simulink model "FRNmodel_IMHRC"  (Simulink 7.9)
settings: Solver=VariableStepDiscrete  StartTime=0.0  StopTime=100.0  RelTol=1e-3
libraries: simeventslib x30
(part 1 of 3)
settings Model: Creator=tsprock3  LastModifiedBy=tsprock3
settings DebuggingCC: SimStateOlderReleaseMsg=warning

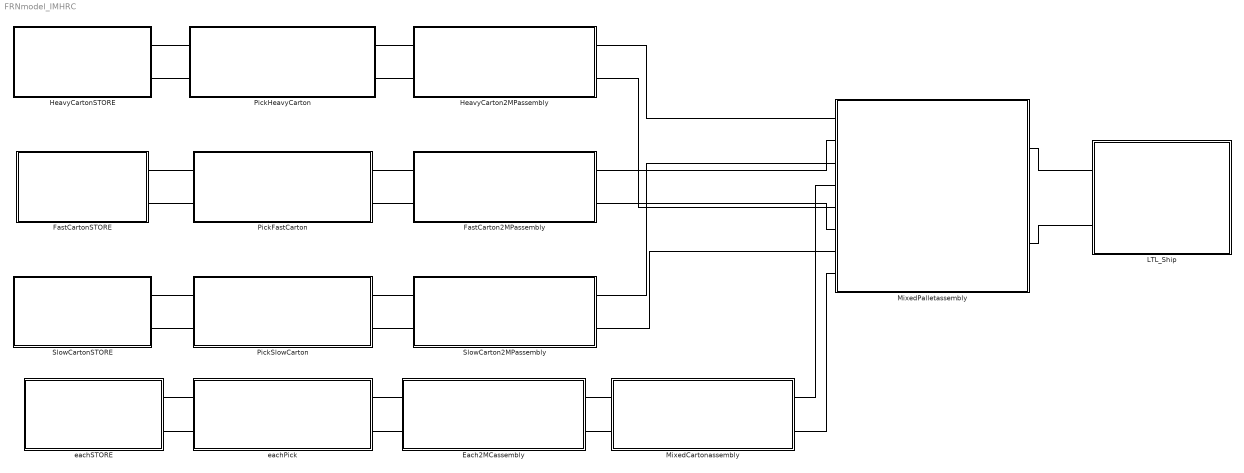
== system FRNmodel_IMHRC ==
  Each2MCassembly : Subsystem
  FastCarton2MPassembly : Subsystem
  FastCartonSTORE : Subsystem
  HeavyCarton2MPassembly : Subsystem
  HeavyCartonSTORE : Subsystem
  LTL_Ship : Subsystem
  MixedCartonassembly : Subsystem
  MixedPalletassembly : Subsystem
  PickFastCarton : Subsystem
  PickHeavyCarton : Subsystem
  PickSlowCarton : Subsystem
  SlowCarton2MPassembly : Subsystem
  SlowCartonSTORE : Subsystem
  eachPick : Subsystem
  eachSTORE : Subsystem
  connections:
  HeavyCartonSTORE/RConn1 -- PickHeavyCarton/LConn1
  FastCartonSTORE/RConn1 -- PickFastCarton/LConn1
  SlowCartonSTORE/RConn1 -- PickSlowCarton/LConn1
  PickHeavyCarton/RConn1 -- HeavyCarton2MPassembly/LConn1
  PickFastCarton/RConn1 -- FastCarton2MPassembly/LConn1
  PickSlowCarton/RConn1 -- SlowCarton2MPassembly/LConn1
  HeavyCarton2MPassembly/RConn1 -- MixedPalletassembly/LConn1
  MixedPalletassembly/RConn1 -- LTL_Ship/LConn1
  FastCarton2MPassembly/RConn1 -- MixedPalletassembly/LConn2
  SlowCarton2MPassembly/RConn1 -- MixedPalletassembly/LConn3
  HeavyCartonSTORE/RConn2 -- PickHeavyCarton/LConn2
  PickFastCarton/LConn2 -- FastCartonSTORE/RConn2
  PickSlowCarton/LConn2 -- SlowCartonSTORE/RConn2
  PickSlowCarton/RConn2 -- SlowCarton2MPassembly/LConn2
  PickFastCarton/RConn2 -- FastCarton2MPassembly/LConn2
  HeavyCarton2MPassembly/LConn2 -- PickHeavyCarton/RConn2
  MixedPalletassembly/LConn5 -- HeavyCarton2MPassembly/RConn2
  MixedPalletassembly/LConn6 -- FastCarton2MPassembly/RConn2
  MixedPalletassembly/LConn7 -- SlowCarton2MPassembly/RConn2
  LTL_Ship/LConn2 -- MixedPalletassembly/RConn2
  Each2MCassembly/RConn1 -- MixedCartonassembly/LConn1
  eachSTORE/RConn1 -- eachPick/LConn1
  eachPick/RConn1 -- Each2MCassembly/LConn1
  eachPick/LConn2 -- eachSTORE/RConn2
  eachPick/RConn2 -- Each2MCassembly/LConn2
  Each2MCassembly/RConn2 -- MixedCartonassembly/LConn2
  MixedPalletassembly/LConn8 -- MixedCartonassembly/RConn2
  MixedPalletassembly/LConn4 -- MixedCartonassembly/RConn1

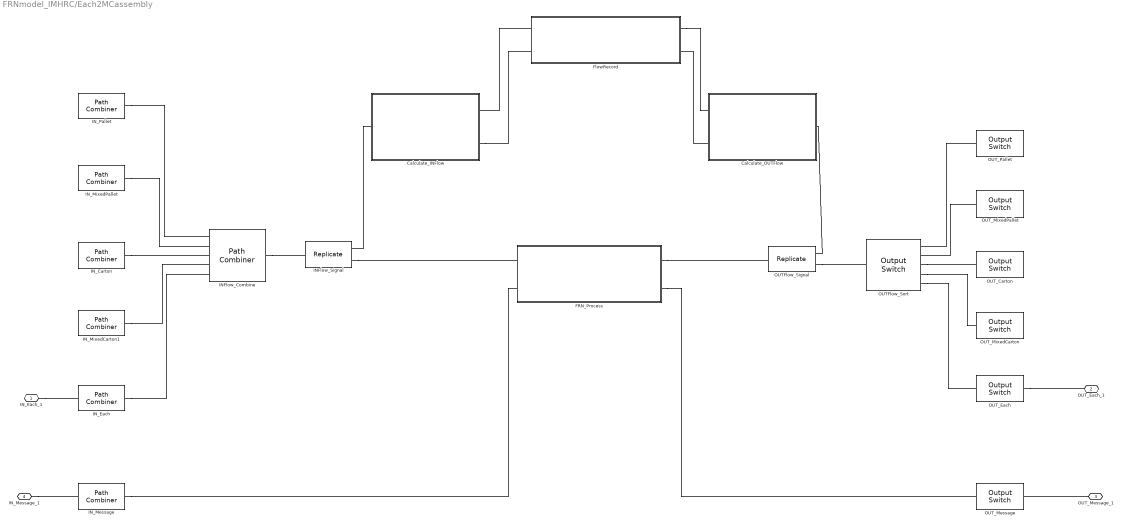
== system FRNmodel_IMHRC/Each2MCassembly ==
  Calculate_INFlow : Subsystem
  Calculate_OUTFlow : Subsystem
  FRN_Process : Subsystem
  FlowRecord : Subsystem
  INFlow_Combine : PathCombiner  NumberInputPorts=5
  INFlow_Signal : Replicate  NumberOutputPorts=2
  IN_Carton : PathCombiner  NumberInputPorts=1
  IN_Each : PathCombiner  NumberInputPorts=1
  IN_Message : PathCombiner  NumberInputPorts=1
  IN_MixedCarton1 : PathCombiner  NumberInputPorts=1
  IN_MixedPallet : PathCombiner  NumberInputPorts=1
  IN_Pallet : PathCombiner  NumberInputPorts=1
  OUTFlow_Signal : Replicate  NumberOutputPorts=2
  OUTFlow_Sort : OutputSwitch  NumberOutputPorts=5  SwitchingCriterion=From attribute  AttributeName=UoH
  OUT_Carton : OutputSwitch  NumberOutputPorts=1
  OUT_Each : OutputSwitch  NumberOutputPorts=1
  OUT_Message : OutputSwitch  NumberOutputPorts=1
  OUT_MixedCarton : OutputSwitch  NumberOutputPorts=1
  OUT_MixedPallet : OutputSwitch  NumberOutputPorts=1
  OUT_Pallet : OutputSwitch  NumberOutputPorts=1
  IN_Each_1 : PMIOPort  Port=1  Side=Left
  OUT_Each_1 : PMIOPort  Port=2  Side=Right
  OUT_Message_1 : PMIOPort  Port=3  Side=Left
  IN_Message_1 : PMIOPort  Port=4  Side=Right
  connections:
  Calculate_INFlow/LConn1 -- INFlow_Signal/RConn1
  FlowRecord/RConn1 -- Calculate_INFlow/RConn1
  Calculate_INFlow/RConn2 -- FlowRecord/RConn2
  FlowRecord/LConn1 -- Calculate_OUTFlow/LConn1
  Calculate_OUTFlow/LConn2 -- FlowRecord/LConn2
  INFlow_Signal/RConn2 -- FRN_Process/LConn1
  FRN_Process/RConn1 -- OUTFlow_Signal/LConn1
  OUTFlow_Signal/RConn1 -- Calculate_OUTFlow/RConn1
  INFlow_Combine/RConn1 -- INFlow_Signal/LConn1
  IN_Pallet/RConn1 -- INFlow_Combine/LConn1
  IN_Carton/RConn1 -- INFlow_Combine/LConn3
  IN_Each/RConn1 -- INFlow_Combine/LConn5
  OUTFlow_Signal/RConn2 -- OUTFlow_Sort/LConn1
  OUT_Pallet/LConn1 -- OUTFlow_Sort/RConn1
  OUTFlow_Sort/RConn3 -- OUT_Carton/LConn1
  OUTFlow_Sort/RConn5 -- OUT_Each/LConn1
  IN_Message_1/RConn1 -- IN_Message/LConn1
  OUT_Message_1/RConn1 -- OUT_Message/RConn1
  IN_Message/RConn1 -- FRN_Process/LConn2
  FRN_Process/RConn2 -- OUT_Message/LConn1
  OUT_MixedPallet/LConn1 -- OUTFlow_Sort/RConn2
  OUTFlow_Sort/RConn4 -- OUT_MixedCarton/LConn1
  IN_MixedPallet/RConn1 -- INFlow_Combine/LConn2
  IN_MixedCarton1/RConn1 -- INFlow_Combine/LConn4
  IN_Each_1/RConn1 -- IN_Each/LConn1
  OUT_Each/RConn1 -- OUT_Each_1/RConn1

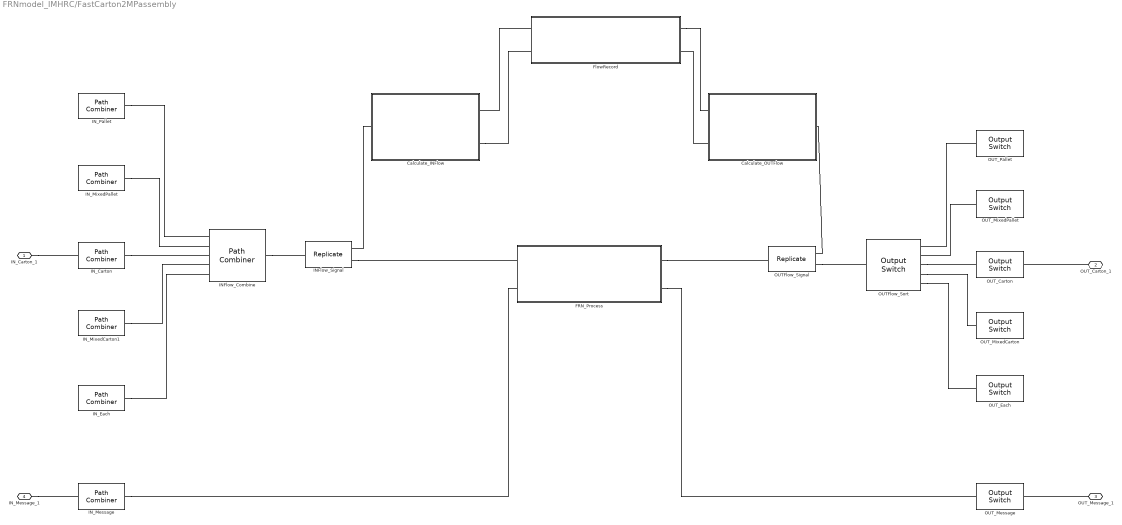
== system FRNmodel_IMHRC/FastCarton2MPassembly ==
  Calculate_INFlow : Subsystem
  Calculate_OUTFlow : Subsystem
  FRN_Process : Subsystem
  FlowRecord : Subsystem
  INFlow_Combine : PathCombiner  NumberInputPorts=5
  INFlow_Signal : Replicate  NumberOutputPorts=2
  IN_Carton : PathCombiner  NumberInputPorts=1
  IN_Each : PathCombiner  NumberInputPorts=1
  IN_Message : PathCombiner  NumberInputPorts=1
  IN_MixedCarton1 : PathCombiner  NumberInputPorts=1
  IN_MixedPallet : PathCombiner  NumberInputPorts=1
  IN_Pallet : PathCombiner  NumberInputPorts=1
  OUTFlow_Signal : Replicate  NumberOutputPorts=2
  OUTFlow_Sort : OutputSwitch  NumberOutputPorts=5  SwitchingCriterion=From attribute  AttributeName=UoH
  OUT_Carton : OutputSwitch  NumberOutputPorts=1
  OUT_Each : OutputSwitch  NumberOutputPorts=1
  OUT_Message : OutputSwitch  NumberOutputPorts=1
  OUT_MixedCarton : OutputSwitch  NumberOutputPorts=1
  OUT_MixedPallet : OutputSwitch  NumberOutputPorts=1
  OUT_Pallet : OutputSwitch  NumberOutputPorts=1
  IN_Carton_1 : PMIOPort  Port=1  Side=Left
  OUT_Carton_1 : PMIOPort  Port=2  Side=Right
  OUT_Message_1 : PMIOPort  Port=3  Side=Left
  IN_Message_1 : PMIOPort  Port=4  Side=Right
  connections:
  Calculate_INFlow/LConn1 -- INFlow_Signal/RConn1
  FlowRecord/RConn1 -- Calculate_INFlow/RConn1
  Calculate_INFlow/RConn2 -- FlowRecord/RConn2
  FlowRecord/LConn1 -- Calculate_OUTFlow/LConn1
  Calculate_OUTFlow/LConn2 -- FlowRecord/LConn2
  INFlow_Signal/RConn2 -- FRN_Process/LConn1
  FRN_Process/RConn1 -- OUTFlow_Signal/LConn1
  OUTFlow_Signal/RConn1 -- Calculate_OUTFlow/RConn1
  INFlow_Combine/RConn1 -- INFlow_Signal/LConn1
  IN_Pallet/RConn1 -- INFlow_Combine/LConn1
  IN_Carton_1/RConn1 -- IN_Carton/LConn1
  IN_Carton/RConn1 -- INFlow_Combine/LConn3
  IN_Each/RConn1 -- INFlow_Combine/LConn5
  OUTFlow_Signal/RConn2 -- OUTFlow_Sort/LConn1
  OUT_Pallet/LConn1 -- OUTFlow_Sort/RConn1
  OUT_Carton_1/RConn1 -- OUT_Carton/RConn1
  OUTFlow_Sort/RConn3 -- OUT_Carton/LConn1
  OUTFlow_Sort/RConn5 -- OUT_Each/LConn1
  IN_Message_1/RConn1 -- IN_Message/LConn1
  OUT_Message_1/RConn1 -- OUT_Message/RConn1
  IN_Message/RConn1 -- FRN_Process/LConn2
  FRN_Process/RConn2 -- OUT_Message/LConn1
  OUT_MixedPallet/LConn1 -- OUTFlow_Sort/RConn2
  OUTFlow_Sort/RConn4 -- OUT_MixedCarton/LConn1
  IN_MixedPallet/RConn1 -- INFlow_Combine/LConn2
  IN_MixedCarton1/RConn1 -- INFlow_Combine/LConn4

== system FRNmodel_IMHRC/FastCartonSTORE ==
  Calculate_INFlow : Subsystem
  Calculate_OUTFlow : Subsystem
  FRN_Process : Subsystem
  FlowRecord : Subsystem
  INFlow_Combine : PathCombiner  NumberInputPorts=5
  INFlow_Signal : Replicate  NumberOutputPorts=2
  IN_Carton : PathCombiner  NumberInputPorts=1
  IN_Each : PathCombiner  NumberInputPorts=1
  IN_Message : PathCombiner  NumberInputPorts=1
  IN_MixedCarton1 : PathCombiner  NumberInputPorts=1
  IN_MixedPallet : PathCombiner  NumberInputPorts=1
  IN_Pallet : PathCombiner  NumberInputPorts=1
  OUTFlow_Signal : Replicate  NumberOutputPorts=2
  OUTFlow_Sort : OutputSwitch  NumberOutputPorts=5  SwitchingCriterion=From attribute  AttributeName=UoH
  OUT_Carton : OutputSwitch  NumberOutputPorts=1
  OUT_Each : OutputSwitch  NumberOutputPorts=1
  OUT_Message : OutputSwitch  NumberOutputPorts=1
  OUT_MixedCarton : OutputSwitch  NumberOutputPorts=1
  OUT_MixedPallet : OutputSwitch  NumberOutputPorts=1
  OUT_Pallet : OutputSwitch  NumberOutputPorts=1
  OUT_Carton_1 : PMIOPort  Port=1  Side=Right
  IN_Message_1 : PMIOPort  Port=2  Side=Right
  connections:
  Calculate_INFlow/LConn1 -- INFlow_Signal/RConn1
  FlowRecord/RConn1 -- Calculate_INFlow/RConn1
  Calculate_INFlow/RConn2 -- FlowRecord/RConn2
  FlowRecord/LConn1 -- Calculate_OUTFlow/LConn1
  Calculate_OUTFlow/LConn2 -- FlowRecord/LConn2
  INFlow_Signal/RConn2 -- FRN_Process/LConn1
  FRN_Process/RConn1 -- OUTFlow_Signal/LConn1
  OUTFlow_Signal/RConn1 -- Calculate_OUTFlow/RConn1
  INFlow_Combine/RConn1 -- INFlow_Signal/LConn1
  IN_Pallet/RConn1 -- INFlow_Combine/LConn1
  IN_Carton/RConn1 -- INFlow_Combine/LConn3
  IN_Each/RConn1 -- INFlow_Combine/LConn5
  OUTFlow_Signal/RConn2 -- OUTFlow_Sort/LConn1
  OUT_Pallet/LConn1 -- OUTFlow_Sort/RConn1
  OUT_Carton_1/RConn1 -- OUT_Carton/RConn1
  OUTFlow_Sort/RConn3 -- OUT_Carton/LConn1
  OUTFlow_Sort/RConn5 -- OUT_Each/LConn1
  IN_Message_1/RConn1 -- IN_Message/LConn1
  IN_Message/RConn1 -- FRN_Process/LConn2
  FRN_Process/RConn2 -- OUT_Message/LConn1
  OUT_MixedPallet/LConn1 -- OUTFlow_Sort/RConn2
  OUTFlow_Sort/RConn4 -- OUT_MixedCarton/LConn1
  IN_MixedPallet/RConn1 -- INFlow_Combine/LConn2
  IN_MixedCarton1/RConn1 -- INFlow_Combine/LConn4

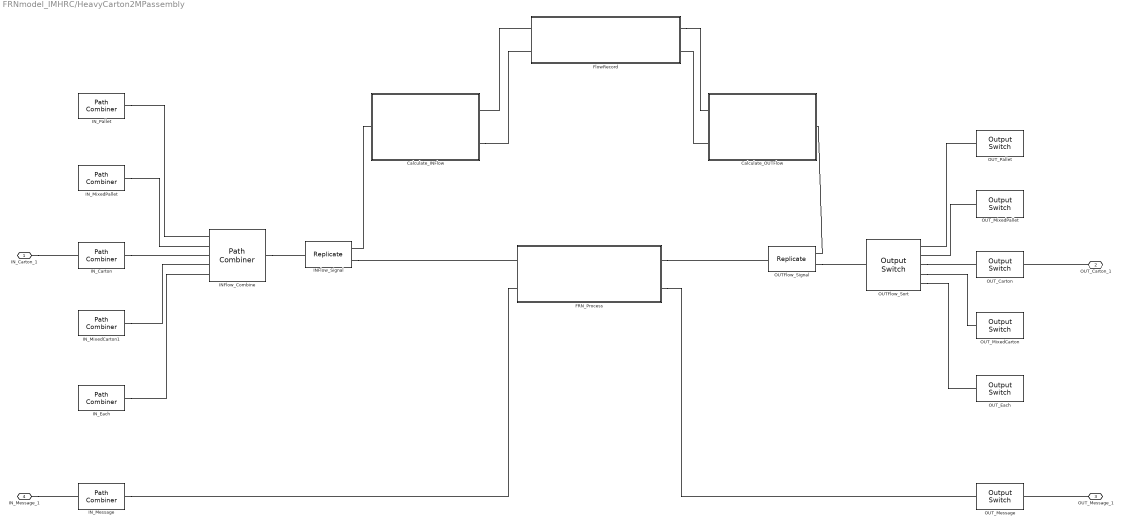
== system FRNmodel_IMHRC/HeavyCarton2MPassembly ==
  Calculate_INFlow : Subsystem
  Calculate_OUTFlow : Subsystem
  FRN_Process : Subsystem
  FlowRecord : Subsystem
  INFlow_Combine : PathCombiner  NumberInputPorts=5
  INFlow_Signal : Replicate  NumberOutputPorts=2
  IN_Carton : PathCombiner  NumberInputPorts=1
  IN_Each : PathCombiner  NumberInputPorts=1
  IN_Message : PathCombiner  NumberInputPorts=1
  IN_MixedCarton1 : PathCombiner  NumberInputPorts=1
  IN_MixedPallet : PathCombiner  NumberInputPorts=1
  IN_Pallet : PathCombiner  NumberInputPorts=1
  OUTFlow_Signal : Replicate  NumberOutputPorts=2
  OUTFlow_Sort : OutputSwitch  NumberOutputPorts=5  SwitchingCriterion=From attribute  AttributeName=UoH
  OUT_Carton : OutputSwitch  NumberOutputPorts=1
  OUT_Each : OutputSwitch  NumberOutputPorts=1
  OUT_Message : OutputSwitch  NumberOutputPorts=1
  OUT_MixedCarton : OutputSwitch  NumberOutputPorts=1
  OUT_MixedPallet : OutputSwitch  NumberOutputPorts=1
  OUT_Pallet : OutputSwitch  NumberOutputPorts=1
  IN_Carton_1 : PMIOPort  Port=1  Side=Left
  OUT_Carton_1 : PMIOPort  Port=2  Side=Right
  OUT_Message_1 : PMIOPort  Port=3  Side=Left
  IN_Message_1 : PMIOPort  Port=4  Side=Right
  connections:
  Calculate_INFlow/LConn1 -- INFlow_Signal/RConn1
  FlowRecord/RConn1 -- Calculate_INFlow/RConn1
  Calculate_INFlow/RConn2 -- FlowRecord/RConn2
  FlowRecord/LConn1 -- Calculate_OUTFlow/LConn1
  Calculate_OUTFlow/LConn2 -- FlowRecord/LConn2
  INFlow_Signal/RConn2 -- FRN_Process/LConn1
  FRN_Process/RConn1 -- OUTFlow_Signal/LConn1
  OUTFlow_Signal/RConn1 -- Calculate_OUTFlow/RConn1
  INFlow_Combine/RConn1 -- INFlow_Signal/LConn1
  IN_Pallet/RConn1 -- INFlow_Combine/LConn1
  IN_Carton_1/RConn1 -- IN_Carton/LConn1
  IN_Carton/RConn1 -- INFlow_Combine/LConn3
  IN_Each/RConn1 -- INFlow_Combine/LConn5
  OUTFlow_Signal/RConn2 -- OUTFlow_Sort/LConn1
  OUT_Pallet/LConn1 -- OUTFlow_Sort/RConn1
  OUT_Carton_1/RConn1 -- OUT_Carton/RConn1
  OUTFlow_Sort/RConn3 -- OUT_Carton/LConn1
  OUTFlow_Sort/RConn5 -- OUT_Each/LConn1
  IN_Message_1/RConn1 -- IN_Message/LConn1
  OUT_Message_1/RConn1 -- OUT_Message/RConn1
  IN_Message/RConn1 -- FRN_Process/LConn2
  FRN_Process/RConn2 -- OUT_Message/LConn1
  OUT_MixedPallet/LConn1 -- OUTFlow_Sort/RConn2
  OUTFlow_Sort/RConn4 -- OUT_MixedCarton/LConn1
  IN_MixedPallet/RConn1 -- INFlow_Combine/LConn2
  IN_MixedCarton1/RConn1 -- INFlow_Combine/LConn4

== system FRNmodel_IMHRC/HeavyCartonSTORE ==
  Calculate_INFlow : Subsystem
  Calculate_OUTFlow : Subsystem
  FRN_Process : Subsystem
  FlowRecord : Subsystem
  INFlow_Combine : PathCombiner  NumberInputPorts=5
  INFlow_Signal : Replicate  NumberOutputPorts=2
  IN_Carton : PathCombiner  NumberInputPorts=1
  IN_Each : PathCombiner  NumberInputPorts=1
  IN_Message : PathCombiner  NumberInputPorts=1
  IN_MixedCarton1 : PathCombiner  NumberInputPorts=1
  IN_MixedPallet : PathCombiner  NumberInputPorts=1
  IN_Pallet : PathCombiner  NumberInputPorts=1
  OUTFlow_Signal : Replicate  NumberOutputPorts=2
  OUTFlow_Sort : OutputSwitch  NumberOutputPorts=5  SwitchingCriterion=From attribute  AttributeName=UoH
  OUT_Carton : OutputSwitch  NumberOutputPorts=1
  OUT_Each : OutputSwitch  NumberOutputPorts=1
  OUT_Message : OutputSwitch  NumberOutputPorts=1
  OUT_MixedCarton : OutputSwitch  NumberOutputPorts=1
  OUT_MixedPallet : OutputSwitch  NumberOutputPorts=1
  OUT_Pallet : OutputSwitch  NumberOutputPorts=1
  OUT_Carton_1 : PMIOPort  Port=1  Side=Right
  IN_Message_1 : PMIOPort  Port=2  Side=Right
  connections:
  Calculate_INFlow/LConn1 -- INFlow_Signal/RConn1
  FlowRecord/RConn1 -- Calculate_INFlow/RConn1
  Calculate_INFlow/RConn2 -- FlowRecord/RConn2
  FlowRecord/LConn1 -- Calculate_OUTFlow/LConn1
  Calculate_OUTFlow/LConn2 -- FlowRecord/LConn2
  INFlow_Signal/RConn2 -- FRN_Process/LConn1
  FRN_Process/RConn1 -- OUTFlow_Signal/LConn1
  OUTFlow_Signal/RConn1 -- Calculate_OUTFlow/RConn1
  INFlow_Combine/RConn1 -- INFlow_Signal/LConn1
  IN_Pallet/RConn1 -- INFlow_Combine/LConn1
  IN_Carton/RConn1 -- INFlow_Combine/LConn3
  IN_Each/RConn1 -- INFlow_Combine/LConn5
  OUTFlow_Signal/RConn2 -- OUTFlow_Sort/LConn1
  OUT_Pallet/LConn1 -- OUTFlow_Sort/RConn1
  OUT_Carton_1/RConn1 -- OUT_Carton/RConn1
  OUTFlow_Sort/RConn3 -- OUT_Carton/LConn1
  OUTFlow_Sort/RConn5 -- OUT_Each/LConn1
  IN_Message_1/RConn1 -- IN_Message/LConn1
  IN_Message/RConn1 -- FRN_Process/LConn2
  FRN_Process/RConn2 -- OUT_Message/LConn1
  OUT_MixedPallet/LConn1 -- OUTFlow_Sort/RConn2
  OUTFlow_Sort/RConn4 -- OUT_MixedCarton/LConn1
  IN_MixedPallet/RConn1 -- INFlow_Combine/LConn2
  IN_MixedCarton1/RConn1 -- INFlow_Combine/LConn4

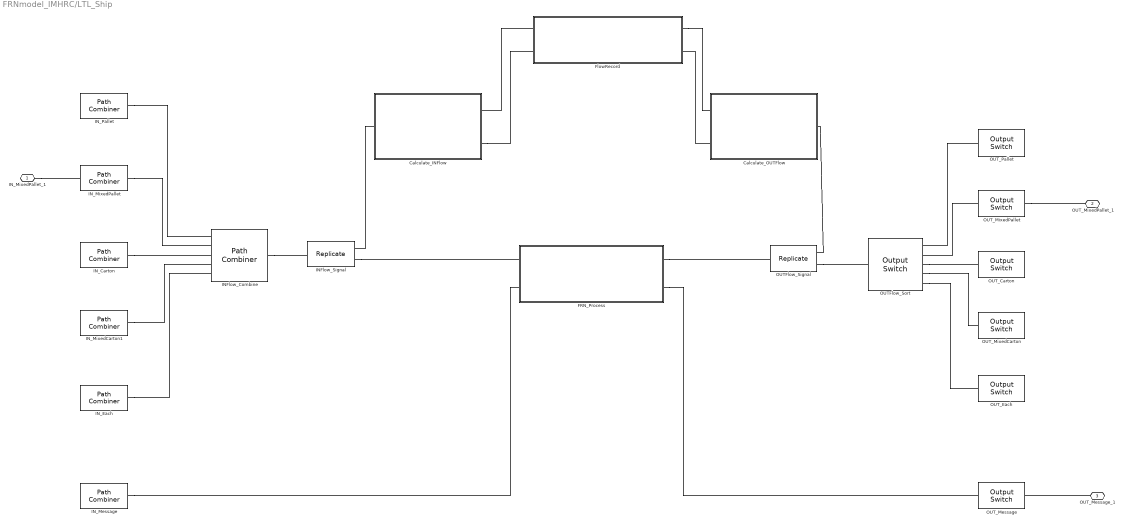
== system FRNmodel_IMHRC/LTL_Ship ==
  Calculate_INFlow : Subsystem
  Calculate_OUTFlow : Subsystem
  FRN_Process : Subsystem
  FlowRecord : Subsystem
  INFlow_Combine : PathCombiner  NumberInputPorts=5
  INFlow_Signal : Replicate  NumberOutputPorts=2
  IN_Carton : PathCombiner  NumberInputPorts=1
  IN_Each : PathCombiner  NumberInputPorts=1
  IN_Message : PathCombiner  NumberInputPorts=1
  IN_MixedCarton1 : PathCombiner  NumberInputPorts=1
  IN_MixedPallet : PathCombiner  NumberInputPorts=1
  IN_Pallet : PathCombiner  NumberInputPorts=1
  OUTFlow_Signal : Replicate  NumberOutputPorts=2
  OUTFlow_Sort : OutputSwitch  NumberOutputPorts=5  SwitchingCriterion=From attribute  AttributeName=UoH
  OUT_Carton : OutputSwitch  NumberOutputPorts=1
  OUT_Each : OutputSwitch  NumberOutputPorts=1
  OUT_Message : OutputSwitch  NumberOutputPorts=1
  OUT_MixedCarton : OutputSwitch  NumberOutputPorts=1
  OUT_MixedPallet : OutputSwitch  NumberOutputPorts=1
  OUT_Pallet : OutputSwitch  NumberOutputPorts=1
  IN_MixedPallet_1 : PMIOPort  Port=1  Side=Left
  OUT_MixedPallet_1 : PMIOPort  Port=2  Side=Right
  OUT_Message_1 : PMIOPort  Port=3  Side=Left
  connections:
  Calculate_INFlow/LConn1 -- INFlow_Signal/RConn1
  FlowRecord/RConn1 -- Calculate_INFlow/RConn1
  Calculate_INFlow/RConn2 -- FlowRecord/RConn2
  FlowRecord/LConn1 -- Calculate_OUTFlow/LConn1
  Calculate_OUTFlow/LConn2 -- FlowRecord/LConn2
  INFlow_Signal/RConn2 -- FRN_Process/LConn1
  FRN_Process/RConn1 -- OUTFlow_Signal/LConn1
  OUTFlow_Signal/RConn1 -- Calculate_OUTFlow/RConn1
  INFlow_Combine/RConn1 -- INFlow_Signal/LConn1
  IN_Pallet/RConn1 -- INFlow_Combine/LConn1
  IN_Carton/RConn1 -- INFlow_Combine/LConn3
  IN_Each/RConn1 -- INFlow_Combine/LConn5
  OUTFlow_Signal/RConn2 -- OUTFlow_Sort/LConn1
  OUT_Pallet/LConn1 -- OUTFlow_Sort/RConn1
  OUTFlow_Sort/RConn3 -- OUT_Carton/LConn1
  OUTFlow_Sort/RConn5 -- OUT_Each/LConn1
  OUT_Message_1/RConn1 -- OUT_Message/RConn1
  IN_Message/RConn1 -- FRN_Process/LConn2
  FRN_Process/RConn2 -- OUT_Message/LConn1
  OUT_MixedPallet/LConn1 -- OUTFlow_Sort/RConn2
  OUTFlow_Sort/RConn4 -- OUT_MixedCarton/LConn1
  IN_MixedPallet/RConn1 -- INFlow_Combine/LConn2
  IN_MixedPallet_1/RConn1 -- IN_MixedPallet/LConn1
  IN_MixedCarton1/RConn1 -- INFlow_Combine/LConn4
  OUT_MixedPallet/RConn1 -- OUT_MixedPallet_1/RConn1

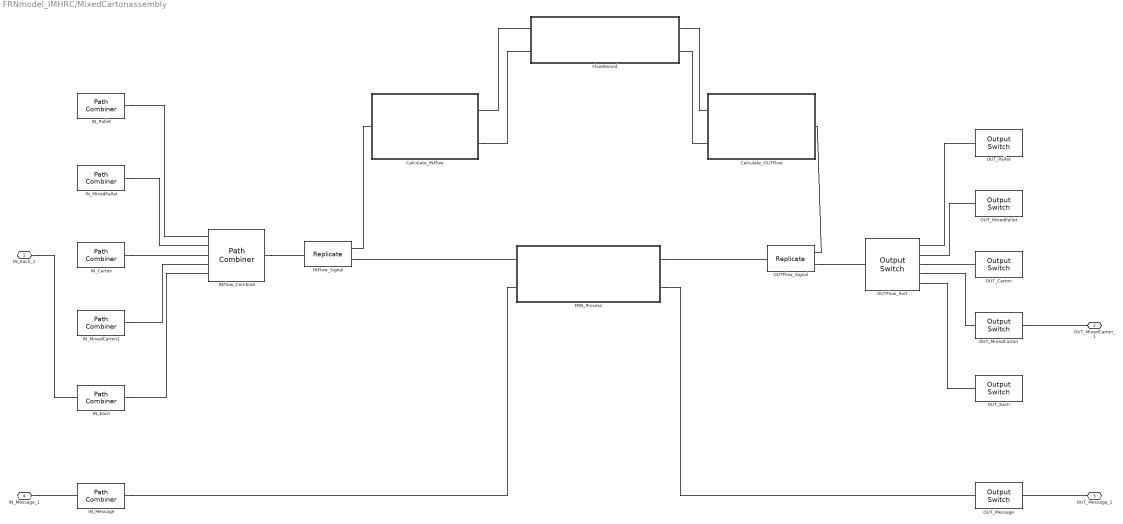
== system FRNmodel_IMHRC/MixedCartonassembly ==
  Calculate_INFlow : Subsystem
  Calculate_OUTFlow : Subsystem
  FRN_Process : Subsystem
  FlowRecord : Subsystem
  INFlow_Combine : PathCombiner  NumberInputPorts=5
  INFlow_Signal : Replicate  NumberOutputPorts=2
  IN_Carton : PathCombiner  NumberInputPorts=1
  IN_Each : PathCombiner  NumberInputPorts=1
  IN_Message : PathCombiner  NumberInputPorts=1
  IN_MixedCarton1 : PathCombiner  NumberInputPorts=1
  IN_MixedPallet : PathCombiner  NumberInputPorts=1
  IN_Pallet : PathCombiner  NumberInputPorts=1
  OUTFlow_Signal : Replicate  NumberOutputPorts=2
  OUTFlow_Sort : OutputSwitch  NumberOutputPorts=5  SwitchingCriterion=From attribute  AttributeName=UoH
  OUT_Carton : OutputSwitch  NumberOutputPorts=1
  OUT_Each : OutputSwitch  NumberOutputPorts=1
  OUT_Message : OutputSwitch  NumberOutputPorts=1
  OUT_MixedCarton : OutputSwitch  NumberOutputPorts=1
  OUT_MixedPallet : OutputSwitch  NumberOutputPorts=1
  OUT_Pallet : OutputSwitch  NumberOutputPorts=1
  IN_Each_1 : PMIOPort  Port=1  Side=Left
  OUT_MixedCarton_1 : PMIOPort  Port=2  Side=Right
  OUT_Message_1 : PMIOPort  Port=3  Side=Left
  IN_Message_1 : PMIOPort  Port=4  Side=Right
  connections:
  Calculate_INFlow/LConn1 -- INFlow_Signal/RConn1
  FlowRecord/RConn1 -- Calculate_INFlow/RConn1
  Calculate_INFlow/RConn2 -- FlowRecord/RConn2
  FlowRecord/LConn1 -- Calculate_OUTFlow/LConn1
  Calculate_OUTFlow/LConn2 -- FlowRecord/LConn2
  INFlow_Signal/RConn2 -- FRN_Process/LConn1
  FRN_Process/RConn1 -- OUTFlow_Signal/LConn1
  OUTFlow_Signal/RConn1 -- Calculate_OUTFlow/RConn1
  INFlow_Combine/RConn1 -- INFlow_Signal/LConn1
  IN_Pallet/RConn1 -- INFlow_Combine/LConn1
  IN_Carton/RConn1 -- INFlow_Combine/LConn3
  IN_Each/RConn1 -- INFlow_Combine/LConn5
  OUTFlow_Signal/RConn2 -- OUTFlow_Sort/LConn1
  OUT_Pallet/LConn1 -- OUTFlow_Sort/RConn1
  OUTFlow_Sort/RConn3 -- OUT_Carton/LConn1
  OUTFlow_Sort/RConn5 -- OUT_Each/LConn1
  IN_Message_1/RConn1 -- IN_Message/LConn1
  OUT_Message_1/RConn1 -- OUT_Message/RConn1
  IN_Message/RConn1 -- FRN_Process/LConn2
  FRN_Process/RConn2 -- OUT_Message/LConn1
  OUT_MixedPallet/LConn1 -- OUTFlow_Sort/RConn2
  OUTFlow_Sort/RConn4 -- OUT_MixedCarton/LConn1
  IN_MixedPallet/RConn1 -- INFlow_Combine/LConn2
  IN_MixedCarton1/RConn1 -- INFlow_Combine/LConn4
  OUT_MixedCarton/RConn1 -- OUT_MixedCarton_1/RConn1
  IN_Each_1/RConn1 -- IN_Each/LConn1

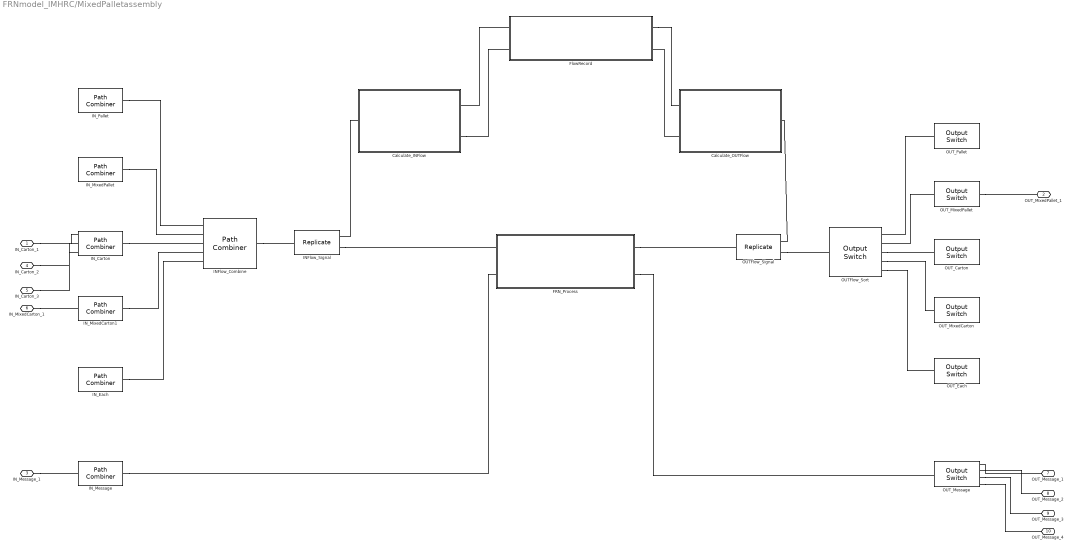
== system FRNmodel_IMHRC/MixedPalletassembly ==
  Calculate_INFlow : Subsystem
  Calculate_OUTFlow : Subsystem
  FRN_Process : Subsystem
  FlowRecord : Subsystem
  INFlow_Combine : PathCombiner  NumberInputPorts=5
  INFlow_Signal : Replicate  NumberOutputPorts=2
  IN_Carton : PathCombiner
  IN_Each : PathCombiner  NumberInputPorts=1
  IN_Message : PathCombiner  NumberInputPorts=1
  IN_MixedCarton1 : PathCombiner  NumberInputPorts=1
  IN_MixedPallet : PathCombiner  NumberInputPorts=1
  IN_Pallet : PathCombiner  NumberInputPorts=1
  OUTFlow_Signal : Replicate  NumberOutputPorts=2
  OUTFlow_Sort : OutputSwitch  NumberOutputPorts=5  SwitchingCriterion=From attribute  AttributeName=UoH
  OUT_Carton : OutputSwitch  NumberOutputPorts=1
  OUT_Each : OutputSwitch  NumberOutputPorts=1
  OUT_Message : OutputSwitch  NumberOutputPorts=4
  OUT_MixedCarton : OutputSwitch  NumberOutputPorts=1
  OUT_MixedPallet : OutputSwitch  NumberOutputPorts=1
  OUT_Pallet : OutputSwitch  NumberOutputPorts=1
  IN_Carton_1 : PMIOPort  Port=1  Side=Left
  OUT_MixedPallet_1 : PMIOPort  Port=2  Side=Right
  IN_Message_1 : PMIOPort  Port=3  Side=Right
  IN_Carton_2 : PMIOPort  Port=4  Side=Left
  IN_Carton_3 : PMIOPort  Port=5  Side=Left
  IN_MixedCarton_1 : PMIOPort  Port=6  Side=Left
  OUT_Message_1 : PMIOPort  Port=7  Side=Left
  OUT_Message_2 : PMIOPort  Port=8  Side=Left
  OUT_Message_3 : PMIOPort  Port=9  Side=Left
  OUT_Message_4 : PMIOPort  Port=10  Side=Left
  connections:
  Calculate_INFlow/LConn1 -- INFlow_Signal/RConn1
  FlowRecord/RConn1 -- Calculate_INFlow/RConn1
  Calculate_INFlow/RConn2 -- FlowRecord/RConn2
  FlowRecord/LConn1 -- Calculate_OUTFlow/LConn1
  Calculate_OUTFlow/LConn2 -- FlowRecord/LConn2
  INFlow_Signal/RConn2 -- FRN_Process/LConn1
  FRN_Process/RConn1 -- OUTFlow_Signal/LConn1
  OUTFlow_Signal/RConn1 -- Calculate_OUTFlow/RConn1
  INFlow_Combine/RConn1 -- INFlow_Signal/LConn1
  IN_Pallet/RConn1 -- INFlow_Combine/LConn1
  IN_Carton_1/RConn1 -- IN_Carton/LConn1
  IN_Carton/RConn1 -- INFlow_Combine/LConn3
  IN_Each/RConn1 -- INFlow_Combine/LConn5
  OUTFlow_Signal/RConn2 -- OUTFlow_Sort/LConn1
  OUT_Pallet/LConn1 -- OUTFlow_Sort/RConn1
  OUTFlow_Sort/RConn3 -- OUT_Carton/LConn1
  OUTFlow_Sort/RConn5 -- OUT_Each/LConn1
  IN_Message_1/RConn1 -- IN_Message/LConn1
  OUT_Message_1/RConn1 -- OUT_Message/RConn1
  IN_Message/RConn1 -- FRN_Process/LConn2
  FRN_Process/RConn2 -- OUT_Message/LConn1
  OUT_MixedPallet/LConn1 -- OUTFlow_Sort/RConn2
  OUTFlow_Sort/RConn4 -- OUT_MixedCarton/LConn1
  IN_MixedPallet/RConn1 -- INFlow_Combine/LConn2
  IN_MixedCarton1/RConn1 -- INFlow_Combine/LConn4
  IN_Carton_2/RConn1 -- IN_Carton/LConn2
  IN_Carton_3/RConn1 -- IN_Carton/LConn3
  OUT_MixedPallet/RConn1 -- OUT_MixedPallet_1/RConn1
  OUT_Message/RConn2 -- OUT_Message_2/RConn1
  OUT_Message/RConn3 -- OUT_Message_3/RConn1
  IN_MixedCarton_1/RConn1 -- IN_MixedCarton1/LConn1
  OUT_Message/RConn4 -- OUT_Message_4/RConn1

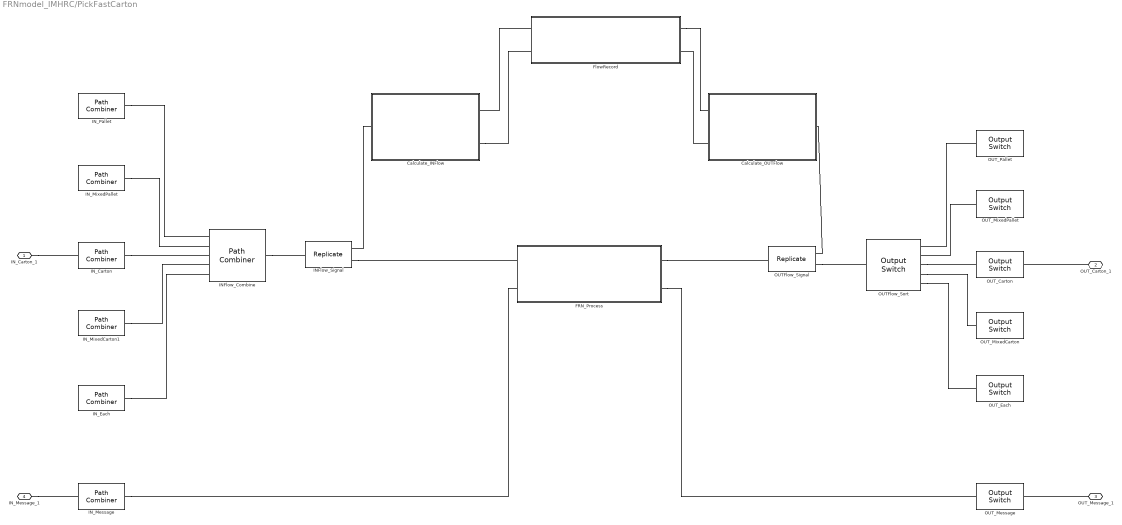
== system FRNmodel_IMHRC/PickFastCarton ==
  Calculate_INFlow : Subsystem
  Calculate_OUTFlow : Subsystem
  FRN_Process : Subsystem
  FlowRecord : Subsystem
  INFlow_Combine : PathCombiner  NumberInputPorts=5
  INFlow_Signal : Replicate  NumberOutputPorts=2
  IN_Carton : PathCombiner  NumberInputPorts=1
  IN_Each : PathCombiner  NumberInputPorts=1
  IN_Message : PathCombiner  NumberInputPorts=1
  IN_MixedCarton1 : PathCombiner  NumberInputPorts=1
  IN_MixedPallet : PathCombiner  NumberInputPorts=1
  IN_Pallet : PathCombiner  NumberInputPorts=1
  OUTFlow_Signal : Replicate  NumberOutputPorts=2
  OUTFlow_Sort : OutputSwitch  NumberOutputPorts=5  SwitchingCriterion=From attribute  AttributeName=UoH
  OUT_Carton : OutputSwitch  NumberOutputPorts=1
  OUT_Each : OutputSwitch  NumberOutputPorts=1
  OUT_Message : OutputSwitch  NumberOutputPorts=1
  OUT_MixedCarton : OutputSwitch  NumberOutputPorts=1
  OUT_MixedPallet : OutputSwitch  NumberOutputPorts=1
  OUT_Pallet : OutputSwitch  NumberOutputPorts=1
  IN_Carton_1 : PMIOPort  Port=1  Side=Left
  OUT_Carton_1 : PMIOPort  Port=2  Side=Right
  OUT_Message_1 : PMIOPort  Port=3  Side=Left
  IN_Message_1 : PMIOPort  Port=4  Side=Right
  connections:
  Calculate_INFlow/LConn1 -- INFlow_Signal/RConn1
  FlowRecord/RConn1 -- Calculate_INFlow/RConn1
  Calculate_INFlow/RConn2 -- FlowRecord/RConn2
  FlowRecord/LConn1 -- Calculate_OUTFlow/LConn1
  Calculate_OUTFlow/LConn2 -- FlowRecord/LConn2
  INFlow_Signal/RConn2 -- FRN_Process/LConn1
  FRN_Process/RConn1 -- OUTFlow_Signal/LConn1
  OUTFlow_Signal/RConn1 -- Calculate_OUTFlow/RConn1
  INFlow_Combine/RConn1 -- INFlow_Signal/LConn1
  IN_Pallet/RConn1 -- INFlow_Combine/LConn1
  IN_Carton_1/RConn1 -- IN_Carton/LConn1
  IN_Carton/RConn1 -- INFlow_Combine/LConn3
  IN_Each/RConn1 -- INFlow_Combine/LConn5
  OUTFlow_Signal/RConn2 -- OUTFlow_Sort/LConn1
  OUT_Pallet/LConn1 -- OUTFlow_Sort/RConn1
  OUT_Carton_1/RConn1 -- OUT_Carton/RConn1
  OUTFlow_Sort/RConn3 -- OUT_Carton/LConn1
  OUTFlow_Sort/RConn5 -- OUT_Each/LConn1
  IN_Message_1/RConn1 -- IN_Message/LConn1
  OUT_Message_1/RConn1 -- OUT_Message/RConn1
  IN_Message/RConn1 -- FRN_Process/LConn2
  FRN_Process/RConn2 -- OUT_Message/LConn1
  OUT_MixedPallet/LConn1 -- OUTFlow_Sort/RConn2
  OUTFlow_Sort/RConn4 -- OUT_MixedCarton/LConn1
  IN_MixedPallet/RConn1 -- INFlow_Combine/LConn2
  IN_MixedCarton1/RConn1 -- INFlow_Combine/LConn4

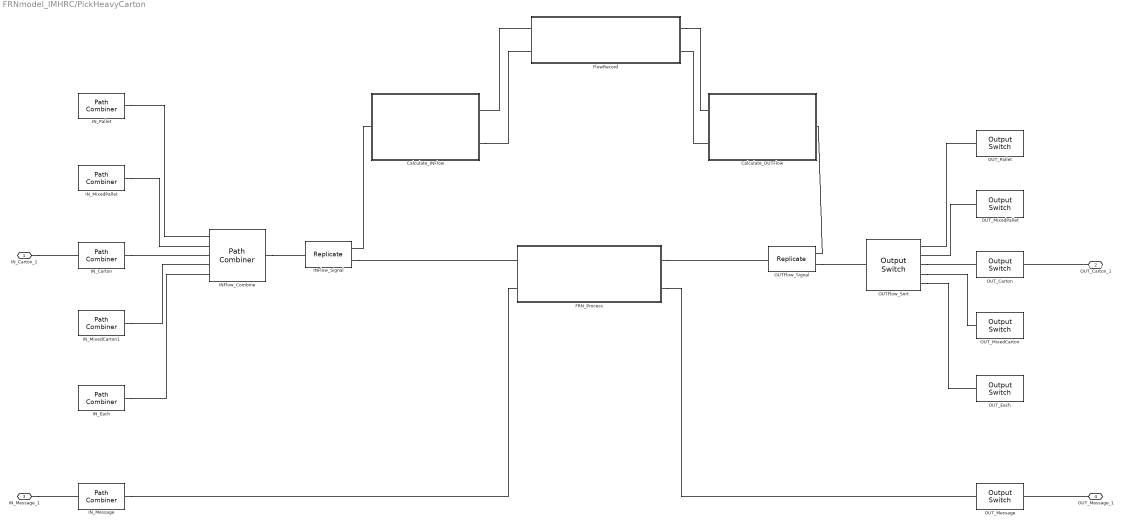
== system FRNmodel_IMHRC/PickHeavyCarton ==
  Calculate_INFlow : Subsystem
  Calculate_OUTFlow : Subsystem
  FRN_Process : Subsystem
  FlowRecord : Subsystem
  INFlow_Combine : PathCombiner  NumberInputPorts=5
  INFlow_Signal : Replicate  NumberOutputPorts=2
  IN_Carton : PathCombiner  NumberInputPorts=1
  IN_Each : PathCombiner  NumberInputPorts=1
  IN_Message : PathCombiner  NumberInputPorts=1
  IN_MixedCarton1 : PathCombiner  NumberInputPorts=1
  IN_MixedPallet : PathCombiner  NumberInputPorts=1
  IN_Pallet : PathCombiner  NumberInputPorts=1
  OUTFlow_Signal : Replicate  NumberOutputPorts=2
  OUTFlow_Sort : OutputSwitch  NumberOutputPorts=5  SwitchingCriterion=From attribute  AttributeName=UoH
  OUT_Carton : OutputSwitch  NumberOutputPorts=1
  OUT_Each : OutputSwitch  NumberOutputPorts=1
  OUT_Message : OutputSwitch  NumberOutputPorts=1
  OUT_MixedCarton : OutputSwitch  NumberOutputPorts=1
  OUT_MixedPallet : OutputSwitch  NumberOutputPorts=1
  OUT_Pallet : OutputSwitch  NumberOutputPorts=1
  IN_Carton_1 : PMIOPort  Port=1  Side=Left
  OUT_Carton_1 : PMIOPort  Port=2  Side=Right
  IN_Message_1 : PMIOPort  Port=3  Side=Right
  OUT_Message_1 : PMIOPort  Port=4  Side=Left
  connections:
  Calculate_INFlow/LConn1 -- INFlow_Signal/RConn1
  FlowRecord/RConn1 -- Calculate_INFlow/RConn1
  Calculate_INFlow/RConn2 -- FlowRecord/RConn2
  FlowRecord/LConn1 -- Calculate_OUTFlow/LConn1
  Calculate_OUTFlow/LConn2 -- FlowRecord/LConn2
  INFlow_Signal/RConn2 -- FRN_Process/LConn1
  FRN_Process/RConn1 -- OUTFlow_Signal/LConn1
  OUTFlow_Signal/RConn1 -- Calculate_OUTFlow/RConn1
  INFlow_Combine/RConn1 -- INFlow_Signal/LConn1
  IN_Pallet/RConn1 -- INFlow_Combine/LConn1
  IN_Carton_1/RConn1 -- IN_Carton/LConn1
  IN_Carton/RConn1 -- INFlow_Combine/LConn3
  IN_Each/RConn1 -- INFlow_Combine/LConn5
  OUTFlow_Signal/RConn2 -- OUTFlow_Sort/LConn1
  OUT_Pallet/LConn1 -- OUTFlow_Sort/RConn1
  OUT_Carton_1/RConn1 -- OUT_Carton/RConn1
  OUTFlow_Sort/RConn3 -- OUT_Carton/LConn1
  OUTFlow_Sort/RConn5 -- OUT_Each/LConn1
  IN_Message_1/RConn1 -- IN_Message/LConn1
  OUT_Message_1/RConn1 -- OUT_Message/RConn1
  IN_Message/RConn1 -- FRN_Process/LConn2
  FRN_Process/RConn2 -- OUT_Message/LConn1
  OUT_MixedPallet/LConn1 -- OUTFlow_Sort/RConn2
  OUTFlow_Sort/RConn4 -- OUT_MixedCarton/LConn1
  IN_MixedPallet/RConn1 -- INFlow_Combine/LConn2
  IN_MixedCarton1/RConn1 -- INFlow_Combine/LConn4

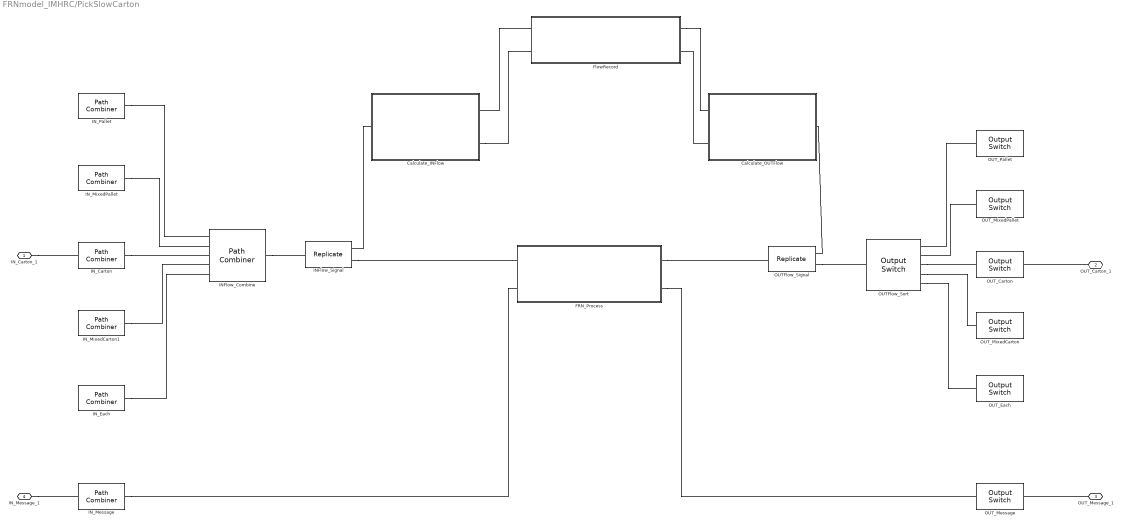
== system FRNmodel_IMHRC/PickSlowCarton ==
  Calculate_INFlow : Subsystem
  Calculate_OUTFlow : Subsystem
  FRN_Process : Subsystem
  FlowRecord : Subsystem
  INFlow_Combine : PathCombiner  NumberInputPorts=5
  INFlow_Signal : Replicate  NumberOutputPorts=2
  IN_Carton : PathCombiner  NumberInputPorts=1
  IN_Each : PathCombiner  NumberInputPorts=1
  IN_Message : PathCombiner  NumberInputPorts=1
  IN_MixedCarton1 : PathCombiner  NumberInputPorts=1
  IN_MixedPallet : PathCombiner  NumberInputPorts=1
  IN_Pallet : PathCombiner  NumberInputPorts=1
  OUTFlow_Signal : Replicate  NumberOutputPorts=2
  OUTFlow_Sort : OutputSwitch  NumberOutputPorts=5  SwitchingCriterion=From attribute  AttributeName=UoH
  OUT_Carton : OutputSwitch  NumberOutputPorts=1
  OUT_Each : OutputSwitch  NumberOutputPorts=1
  OUT_Message : OutputSwitch  NumberOutputPorts=1
  OUT_MixedCarton : OutputSwitch  NumberOutputPorts=1
  OUT_MixedPallet : OutputSwitch  NumberOutputPorts=1
  OUT_Pallet : OutputSwitch  NumberOutputPorts=1
  IN_Carton_1 : PMIOPort  Port=1  Side=Left
  OUT_Carton_1 : PMIOPort  Port=2  Side=Right
  OUT_Message_1 : PMIOPort  Port=3  Side=Left
  IN_Message_1 : PMIOPort  Port=4  Side=Right
  connections:
  Calculate_INFlow/LConn1 -- INFlow_Signal/RConn1
  FlowRecord/RConn1 -- Calculate_INFlow/RConn1
  Calculate_INFlow/RConn2 -- FlowRecord/RConn2
  FlowRecord/LConn1 -- Calculate_OUTFlow/LConn1
  Calculate_OUTFlow/LConn2 -- FlowRecord/LConn2
  INFlow_Signal/RConn2 -- FRN_Process/LConn1
  FRN_Process/RConn1 -- OUTFlow_Signal/LConn1
  OUTFlow_Signal/RConn1 -- Calculate_OUTFlow/RConn1
  INFlow_Combine/RConn1 -- INFlow_Signal/LConn1
  IN_Pallet/RConn1 -- INFlow_Combine/LConn1
  IN_Carton_1/RConn1 -- IN_Carton/LConn1
  IN_Carton/RConn1 -- INFlow_Combine/LConn3
  IN_Each/RConn1 -- INFlow_Combine/LConn5
  OUTFlow_Signal/RConn2 -- OUTFlow_Sort/LConn1
  OUT_Pallet/LConn1 -- OUTFlow_Sort/RConn1
  OUT_Carton_1/RConn1 -- OUT_Carton/RConn1
  OUTFlow_Sort/RConn3 -- OUT_Carton/LConn1
  OUTFlow_Sort/RConn5 -- OUT_Each/LConn1
  IN_Message_1/RConn1 -- IN_Message/LConn1
  OUT_Message_1/RConn1 -- OUT_Message/RConn1
  IN_Message/RConn1 -- FRN_Process/LConn2
  FRN_Process/RConn2 -- OUT_Message/LConn1
  OUT_MixedPallet/LConn1 -- OUTFlow_Sort/RConn2
  OUTFlow_Sort/RConn4 -- OUT_MixedCarton/LConn1
  IN_MixedPallet/RConn1 -- INFlow_Combine/LConn2
  IN_MixedCarton1/RConn1 -- INFlow_Combine/LConn4

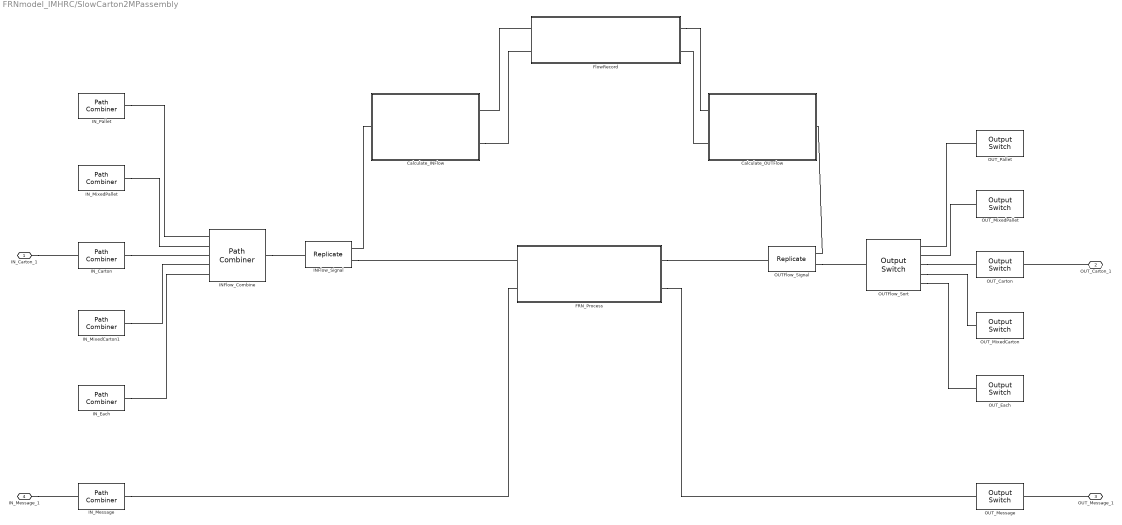
== system FRNmodel_IMHRC/SlowCarton2MPassembly ==
  Calculate_INFlow : Subsystem
  Calculate_OUTFlow : Subsystem
  FRN_Process : Subsystem
  FlowRecord : Subsystem
  INFlow_Combine : PathCombiner  NumberInputPorts=5
  INFlow_Signal : Replicate  NumberOutputPorts=2
  IN_Carton : PathCombiner  NumberInputPorts=1
  IN_Each : PathCombiner  NumberInputPorts=1
  IN_Message : PathCombiner  NumberInputPorts=1
  IN_MixedCarton1 : PathCombiner  NumberInputPorts=1
  IN_MixedPallet : PathCombiner  NumberInputPorts=1
  IN_Pallet : PathCombiner  NumberInputPorts=1
  OUTFlow_Signal : Replicate  NumberOutputPorts=2
  OUTFlow_Sort : OutputSwitch  NumberOutputPorts=5  SwitchingCriterion=From attribute  AttributeName=UoH
  OUT_Carton : OutputSwitch  NumberOutputPorts=1
  OUT_Each : OutputSwitch  NumberOutputPorts=1
  OUT_Message : OutputSwitch  NumberOutputPorts=1
  OUT_MixedCarton : OutputSwitch  NumberOutputPorts=1
  OUT_MixedPallet : OutputSwitch  NumberOutputPorts=1
  OUT_Pallet : OutputSwitch  NumberOutputPorts=1
  IN_Carton_1 : PMIOPort  Port=1  Side=Left
  OUT_Carton_1 : PMIOPort  Port=2  Side=Right
  OUT_Message_1 : PMIOPort  Port=3  Side=Left
  IN_Message_1 : PMIOPort  Port=4  Side=Right
  connections:
  Calculate_INFlow/LConn1 -- INFlow_Signal/RConn1
  FlowRecord/RConn1 -- Calculate_INFlow/RConn1
  Calculate_INFlow/RConn2 -- FlowRecord/RConn2
  FlowRecord/LConn1 -- Calculate_OUTFlow/LConn1
  Calculate_OUTFlow/LConn2 -- FlowRecord/LConn2
  INFlow_Signal/RConn2 -- FRN_Process/LConn1
  FRN_Process/RConn1 -- OUTFlow_Signal/LConn1
  OUTFlow_Signal/RConn1 -- Calculate_OUTFlow/RConn1
  INFlow_Combine/RConn1 -- INFlow_Signal/LConn1
  IN_Pallet/RConn1 -- INFlow_Combine/LConn1
  IN_Carton_1/RConn1 -- IN_Carton/LConn1
  IN_Carton/RConn1 -- INFlow_Combine/LConn3
  IN_Each/RConn1 -- INFlow_Combine/LConn5
  OUTFlow_Signal/RConn2 -- OUTFlow_Sort/LConn1
  OUT_Pallet/LConn1 -- OUTFlow_Sort/RConn1
  OUT_Carton_1/RConn1 -- OUT_Carton/RConn1
  OUTFlow_Sort/RConn3 -- OUT_Carton/LConn1
  OUTFlow_Sort/RConn5 -- OUT_Each/LConn1
  IN_Message_1/RConn1 -- IN_Message/LConn1
  OUT_Message_1/RConn1 -- OUT_Message/RConn1
  IN_Message/RConn1 -- FRN_Process/LConn2
  FRN_Process/RConn2 -- OUT_Message/LConn1
  OUT_MixedPallet/LConn1 -- OUTFlow_Sort/RConn2
  OUTFlow_Sort/RConn4 -- OUT_MixedCarton/LConn1
  IN_MixedPallet/RConn1 -- INFlow_Combine/LConn2
  IN_MixedCarton1/RConn1 -- INFlow_Combine/LConn4

== system FRNmodel_IMHRC/SlowCartonSTORE ==
  Calculate_INFlow : Subsystem
  Calculate_OUTFlow : Subsystem
  FRN_Process : Subsystem
  FlowRecord : Subsystem
  INFlow_Combine : PathCombiner  NumberInputPorts=5
  INFlow_Signal : Replicate  NumberOutputPorts=2
  IN_Carton : PathCombiner  NumberInputPorts=1
  IN_Each : PathCombiner  NumberInputPorts=1
  IN_Message : PathCombiner  NumberInputPorts=1
  IN_MixedCarton1 : PathCombiner  NumberInputPorts=1
  IN_MixedPallet : PathCombiner  NumberInputPorts=1
  IN_Pallet : PathCombiner  NumberInputPorts=1
  OUTFlow_Signal : Replicate  NumberOutputPorts=2
  OUTFlow_Sort : OutputSwitch  NumberOutputPorts=5  SwitchingCriterion=From attribute  AttributeName=UoH
  OUT_Carton : OutputSwitch  NumberOutputPorts=1
  OUT_Each : OutputSwitch  NumberOutputPorts=1
  OUT_Message : OutputSwitch  NumberOutputPorts=1
  OUT_MixedCarton : OutputSwitch  NumberOutputPorts=1
  OUT_MixedPallet : OutputSwitch  NumberOutputPorts=1
  OUT_Pallet : OutputSwitch  NumberOutputPorts=1
  OUT_Carton_1 : PMIOPort  Port=1  Side=Right
  IN_Message_1 : PMIOPort  Port=2  Side=Right
  connections:
  Calculate_INFlow/LConn1 -- INFlow_Signal/RConn1
  FlowRecord/RConn1 -- Calculate_INFlow/RConn1
  Calculate_INFlow/RConn2 -- FlowRecord/RConn2
  FlowRecord/LConn1 -- Calculate_OUTFlow/LConn1
  Calculate_OUTFlow/LConn2 -- FlowRecord/LConn2
  INFlow_Signal/RConn2 -- FRN_Process/LConn1
  FRN_Process/RConn1 -- OUTFlow_Signal/LConn1
  OUTFlow_Signal/RConn1 -- Calculate_OUTFlow/RConn1
  INFlow_Combine/RConn1 -- INFlow_Signal/LConn1
  IN_Pallet/RConn1 -- INFlow_Combine/LConn1
  IN_Carton/RConn1 -- INFlow_Combine/LConn3
  IN_Each/RConn1 -- INFlow_Combine/LConn5
  OUTFlow_Signal/RConn2 -- OUTFlow_Sort/LConn1
  OUT_Pallet/LConn1 -- OUTFlow_Sort/RConn1
  OUT_Carton_1/RConn1 -- OUT_Carton/RConn1
  OUTFlow_Sort/RConn3 -- OUT_Carton/LConn1
  OUTFlow_Sort/RConn5 -- OUT_Each/LConn1
  IN_Message_1/RConn1 -- IN_Message/LConn1
  IN_Message/RConn1 -- FRN_Process/LConn2
  FRN_Process/RConn2 -- OUT_Message/LConn1
  OUT_MixedPallet/LConn1 -- OUTFlow_Sort/RConn2
  OUTFlow_Sort/RConn4 -- OUT_MixedCarton/LConn1
  IN_MixedPallet/RConn1 -- INFlow_Combine/LConn2
  IN_MixedCarton1/RConn1 -- INFlow_Combine/LConn4

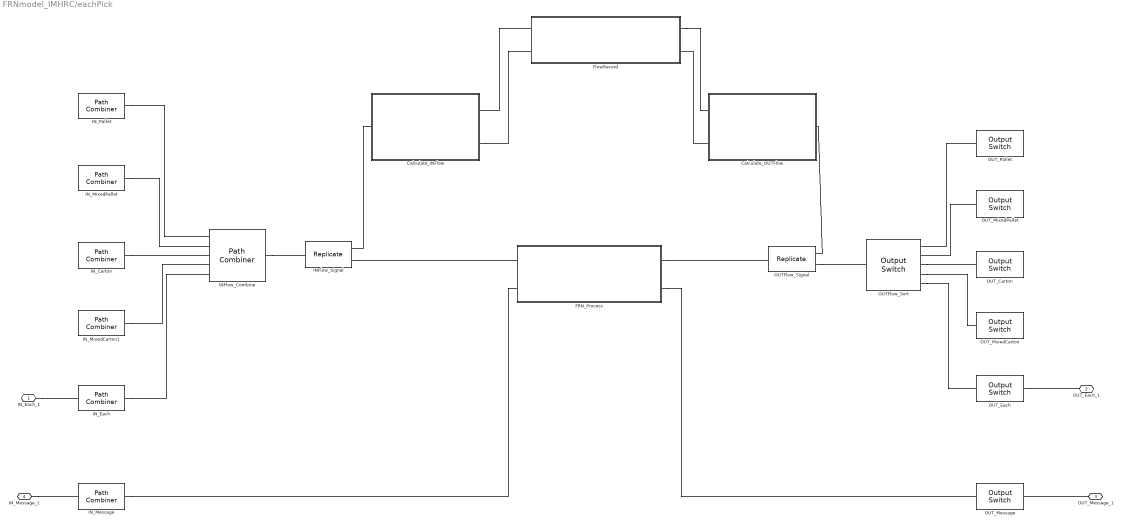
== system FRNmodel_IMHRC/eachPick ==
  Calculate_INFlow : Subsystem
  Calculate_OUTFlow : Subsystem
  FRN_Process : Subsystem
  FlowRecord : Subsystem
  INFlow_Combine : PathCombiner  NumberInputPorts=5
  INFlow_Signal : Replicate  NumberOutputPorts=2
  IN_Carton : PathCombiner  NumberInputPorts=1
  IN_Each : PathCombiner  NumberInputPorts=1
  IN_Message : PathCombiner  NumberInputPorts=1
  IN_MixedCarton1 : PathCombiner  NumberInputPorts=1
  IN_MixedPallet : PathCombiner  NumberInputPorts=1
  IN_Pallet : PathCombiner  NumberInputPorts=1
  OUTFlow_Signal : Replicate  NumberOutputPorts=2
  OUTFlow_Sort : OutputSwitch  NumberOutputPorts=5  SwitchingCriterion=From attribute  AttributeName=UoH
  OUT_Carton : OutputSwitch  NumberOutputPorts=1
  OUT_Each : OutputSwitch  NumberOutputPorts=1
  OUT_Message : OutputSwitch  NumberOutputPorts=1
  OUT_MixedCarton : OutputSwitch  NumberOutputPorts=1
  OUT_MixedPallet : OutputSwitch  NumberOutputPorts=1
  OUT_Pallet : OutputSwitch  NumberOutputPorts=1
  IN_Each_1 : PMIOPort  Port=1  Side=Left
  OUT_Each_1 : PMIOPort  Port=2  Side=Right
  OUT_Message_1 : PMIOPort  Port=3  Side=Left
  IN_Message_1 : PMIOPort  Port=4  Side=Right
  connections:
  Calculate_INFlow/LConn1 -- INFlow_Signal/RConn1
  FlowRecord/RConn1 -- Calculate_INFlow/RConn1
  Calculate_INFlow/RConn2 -- FlowRecord/RConn2
  FlowRecord/LConn1 -- Calculate_OUTFlow/LConn1
  Calculate_OUTFlow/LConn2 -- FlowRecord/LConn2
  INFlow_Signal/RConn2 -- FRN_Process/LConn1
  FRN_Process/RConn1 -- OUTFlow_Signal/LConn1
  OUTFlow_Signal/RConn1 -- Calculate_OUTFlow/RConn1
  INFlow_Combine/RConn1 -- INFlow_Signal/LConn1
  IN_Pallet/RConn1 -- INFlow_Combine/LConn1
  IN_Carton/RConn1 -- INFlow_Combine/LConn3
  IN_Each/RConn1 -- INFlow_Combine/LConn5
  OUTFlow_Signal/RConn2 -- OUTFlow_Sort/LConn1
  OUT_Pallet/LConn1 -- OUTFlow_Sort/RConn1
  OUTFlow_Sort/RConn3 -- OUT_Carton/LConn1
  OUTFlow_Sort/RConn5 -- OUT_Each/LConn1
  IN_Message_1/RConn1 -- IN_Message/LConn1
  OUT_Message_1/RConn1 -- OUT_Message/RConn1
  IN_Message/RConn1 -- FRN_Process/LConn2
  FRN_Process/RConn2 -- OUT_Message/LConn1
  OUT_MixedPallet/LConn1 -- OUTFlow_Sort/RConn2
  OUTFlow_Sort/RConn4 -- OUT_MixedCarton/LConn1
  IN_MixedPallet/RConn1 -- INFlow_Combine/LConn2
  IN_MixedCarton1/RConn1 -- INFlow_Combine/LConn4
  IN_Each_1/RConn1 -- IN_Each/LConn1
  OUT_Each/RConn1 -- OUT_Each_1/RConn1

== system FRNmodel_IMHRC/eachSTORE ==
  Calculate_INFlow : Subsystem
  Calculate_OUTFlow : Subsystem
  FRN_Process : Subsystem
  FlowRecord : Subsystem
  INFlow_Combine : PathCombiner  NumberInputPorts=5
  INFlow_Signal : Replicate  NumberOutputPorts=2
  IN_Carton : PathCombiner  NumberInputPorts=1
  IN_Each : PathCombiner  NumberInputPorts=1
  IN_Message : PathCombiner  NumberInputPorts=1
  IN_MixedCarton1 : PathCombiner  NumberInputPorts=1
  IN_MixedPallet : PathCombiner  NumberInputPorts=1
  IN_Pallet : PathCombiner  NumberInputPorts=1
  OUTFlow_Signal : Replicate  NumberOutputPorts=2
  OUTFlow_Sort : OutputSwitch  NumberOutputPorts=5  SwitchingCriterion=From attribute  AttributeName=UoH
  OUT_Carton : OutputSwitch  NumberOutputPorts=1
  OUT_Each : OutputSwitch  NumberOutputPorts=1
  OUT_Message : OutputSwitch  NumberOutputPorts=1
  OUT_MixedCarton : OutputSwitch  NumberOutputPorts=1
  OUT_MixedPallet : OutputSwitch  NumberOutputPorts=1
  OUT_Pallet : OutputSwitch  NumberOutputPorts=1
  OUT_Each_1 : PMIOPort  Port=1  Side=Right
  IN_Message_1 : PMIOPort  Port=2  Side=Right
  connections:
  Calculate_INFlow/LConn1 -- INFlow_Signal/RConn1
  FlowRecord/RConn1 -- Calculate_INFlow/RConn1
  Calculate_INFlow/RConn2 -- FlowRecord/RConn2
  FlowRecord/LConn1 -- Calculate_OUTFlow/LConn1
  Calculate_OUTFlow/LConn2 -- FlowRecord/LConn2
  INFlow_Signal/RConn2 -- FRN_Process/LConn1
  FRN_Process/RConn1 -- OUTFlow_Signal/LConn1
  OUTFlow_Signal/RConn1 -- Calculate_OUTFlow/RConn1
  INFlow_Combine/RConn1 -- INFlow_Signal/LConn1
  IN_Pallet/RConn1 -- INFlow_Combine/LConn1
  IN_Carton/RConn1 -- INFlow_Combine/LConn3
  IN_Each/RConn1 -- INFlow_Combine/LConn5
  OUTFlow_Signal/RConn2 -- OUTFlow_Sort/LConn1
  OUT_Pallet/LConn1 -- OUTFlow_Sort/RConn1
  OUTFlow_Sort/RConn3 -- OUT_Carton/LConn1
  OUTFlow_Sort/RConn5 -- OUT_Each/LConn1
  IN_Message_1/RConn1 -- IN_Message/LConn1
  IN_Message/RConn1 -- FRN_Process/LConn2
  FRN_Process/RConn2 -- OUT_Message/LConn1
  OUT_MixedPallet/LConn1 -- OUTFlow_Sort/RConn2
  OUTFlow_Sort/RConn4 -- OUT_MixedCarton/LConn1
  IN_MixedPallet/RConn1 -- INFlow_Combine/LConn2
  IN_MixedCarton1/RConn1 -- INFlow_Combine/LConn4
  OUT_Each/RConn1 -- OUT_Each_1/RConn1

== system FRNmodel_IMHRC/Each2MCassembly/Calculate_INFlow ==
  Calculate_INFlow : MATLAB Function  TreatAsAtomicUnit=on
  Entity Combiner : EntityCombiner  NumberInputPorts=2
  Entity Sink : EntitySink
  Entity Splitter : EntitySplitter  NumberOutputPorts=2
  FIFO Queue : FIFOQueue  Capacity=inf
  Get Attribute : GetAttribute  AttributeName=UoH|Quantity|INFlow  AttributeMissing=Error|Error|Error  AttributeDefaultValue=1|1|1  AttributeTreatAsVector=1|1|1  AttributeSendTiming=After entity departure|After entity departure|After entity departure  EvaluatedDefaultAttributeValue={[];[];[]}
      settings: OutputPortMap=o1,o2,o3
  Set Attribute : SetAttribute  AttributeName=INFlow  AttributeFrom=Signal port  EvaluatedAttributeValue={[]}
  Single Server : SingleServer  ServiceTime=0
  FlowRecord_IN : PMIOPort  Port=1  Side=Right
  FlowRecord_OUT : PMIOPort  Port=2  Side=Right
  INFlow_Signal : PMIOPort  Port=3  Side=Left
  wires:
  Get Attribute/1 -> Calculate_INFlow/1(UoH)
  Calculate_INFlow/1(INFlow_return) -> Set Attribute/1
  Get Attribute/2 -> Calculate_INFlow/2(Quantity)
  Get Attribute/3 -> Calculate_INFlow/3(INFlow)
  connections:
  Entity Combiner/RConn1 -- Get Attribute/LConn1
  Set Attribute/RConn1 -- Entity Splitter/LConn1
  Get Attribute/RConn1 -- Single Server/LConn1
  Single Server/RConn1 -- Set Attribute/LConn1
  FlowRecord_OUT/RConn1 -- Entity Splitter/RConn1
  FlowRecord_IN/RConn1 -- Entity Combiner/LConn1
  Entity Splitter/RConn2 -- Entity Sink/LConn1
  INFlow_Signal/RConn1 -- FIFO Queue/LConn1
  FIFO Queue/RConn1 -- Entity Combiner/LConn2

== system FRNmodel_IMHRC/Each2MCassembly/Calculate_OUTFlow ==
  Calculate_OUTFlow : MATLAB Function  TreatAsAtomicUnit=on
  Entity Combiner : EntityCombiner  NumberInputPorts=2
  Entity Sink : EntitySink
  Entity Splitter : EntitySplitter  NumberOutputPorts=2
  FIFO Queue : FIFOQueue  Capacity=inf
  Get Attribute : GetAttribute  AttributeName=UoH|Quantity|OUTFlow  AttributeMissing=Error|Error|Error  AttributeDefaultValue=1|1|1  AttributeTreatAsVector=1|1|1  AttributeSendTiming=After entity departure|After entity departure|After entity departure  EvaluatedDefaultAttributeValue={[];[];[]}
      settings: OutputPortMap=o1,o2,o3
  Set Attribute : SetAttribute  AttributeName=OUTFlow  AttributeFrom=Signal port  EvaluatedAttributeValue={[]}
  Single Server : SingleServer  ServiceTime=0
  FlowRecord_IN : PMIOPort  Port=1  Side=Left
  FlowRecord_OUT : PMIOPort  Port=2  Side=Left
  OUTFlow_Signal : PMIOPort  Port=3  Side=Right
  wires:
  Get Attribute/1 -> Calculate_OUTFlow/1(UoH)
  Calculate_OUTFlow/1(OUTFlow_return) -> Set Attribute/1
  Get Attribute/2 -> Calculate_OUTFlow/2(Quantity)
  Get Attribute/3 -> Calculate_OUTFlow/3(OUTFlow)
  connections:
  Entity Combiner/RConn1 -- Get Attribute/LConn1
  Set Attribute/RConn1 -- Entity Splitter/LConn1
  Get Attribute/RConn1 -- Single Server/LConn1
  Single Server/RConn1 -- Set Attribute/LConn1
  FlowRecord_OUT/RConn1 -- Entity Splitter/RConn1
  FlowRecord_IN/RConn1 -- Entity Combiner/LConn1
  OUTFlow_Signal/RConn1 -- FIFO Queue/LConn1
  FIFO Queue/RConn1 -- Entity Combiner/LConn2
  Entity Splitter/RConn2 -- Entity Sink/LConn1

== system FRNmodel_IMHRC/Each2MCassembly/FRN_Process ==
  FIFO Queue1 : FIFOQueue
  N-Server : NServer  NumberOfServers=inf  ServiceTime=0
  Flow_IN : PMIOPort  Port=1  Side=Left
  Message_IN : PMIOPort  Port=2  Side=Left
  Flow_OUT : PMIOPort  Port=3  Side=Right
  Message_OUT : PMIOPort  Port=4  Side=Right
  connections:
  FIFO Queue1/RConn1 -- N-Server/LConn1
  Flow_IN/RConn1 -- FIFO Queue1/LConn1
  Flow_OUT/RConn1 -- N-Server/RConn1
  Message_OUT/RConn1 -- Message_IN/RConn1

== system FRNmodel_IMHRC/Each2MCassembly/FlowRecord ==
  Discrete Event Signal to Workspace : simeventslib/SimEvents Sinks/Discrete Event Signal to Workspace  VariableName=INFlow_Metric  SaveFormat=Structure With Time  isMonitorOnly=off  isRecordIC=off
  Discrete Event Signal to Workspace1 : simeventslib/SimEvents Sinks/Discrete Event Signal to Workspace  VariableName=OUTFlow_Metric  SaveFormat=Structure With Time  isMonitorOnly=off  isRecordIC=off
  FIFO Queue : FIFOQueue
  FlowRecord : TimeBasedFunctionCallGenerator  EventGenerationMode=Only at simulation start
  Get Attribute : GetAttribute  AttributeName=OUTFlow|INFlow  AttributeMissing=Error|Error  AttributeDefaultValue=1|1  AttributeTreatAsVector=1|1  AttributeSendTiming=After entity departure|After entity departure  EvaluatedDefaultAttributeValue={[];[]}
      settings: OutputPortMap=o1,o2
  Initialize_FlowRecord : SetAttribute  AttributeName=INFlow|OUTFlow  AttributeFrom=Dialog|Dialog  AttributeValue=[0 0 0 0 0]|[0 0 0 0 0]  AttributeTreatAsVector=1|1  EvaluatedAttributeValue={[0 0 0 0 0];[0 0 0 0 0]}
  New_FlowRecord : EventBasedEntityGenerator  GenerateEntitiesUpon=Function call from port fcn
  Output Switch : OutputSwitch  NumberOutputPorts=2
  Path Combiner1 : PathCombiner
  TO_INFlow : PMIOPort  Port=1  Side=Right
  TO_OUTFlow : PMIOPort  Port=2  Side=Left
  FROM_INFlow : PMIOPort  Port=3  Side=Right
  FROM_OUTFlow : PMIOPort  Port=4  Side=Left
  wires:
  FlowRecord/1 -> New_FlowRecord/1
  Get Attribute/2 -> Discrete Event Signal to Workspace/1
  Get Attribute/1 -> Discrete Event Signal to Workspace1/1
  connections:
  Output Switch/LConn1 -- FIFO Queue/RConn1
  New_FlowRecord/RConn1 -- Initialize_FlowRecord/LConn1
  Initialize_FlowRecord/RConn1 -- Path Combiner1/LConn1
  TO_INFlow/RConn1 -- Output Switch/RConn1
  TO_OUTFlow/RConn1 -- Output Switch/RConn2
  FROM_INFlow/RConn1 -- Path Combiner1/LConn2
  FROM_OUTFlow/RConn1 -- Path Combiner1/LConn3
  Path Combiner1/RConn1 -- Get Attribute/LConn1
  Get Attribute/RConn1 -- FIFO Queue/LConn1

== system FRNmodel_IMHRC/FastCarton2MPassembly/Calculate_INFlow ==
  Calculate_INFlow : MATLAB Function  TreatAsAtomicUnit=on
  Entity Combiner : EntityCombiner  NumberInputPorts=2
  Entity Sink : EntitySink
  Entity Splitter : EntitySplitter  NumberOutputPorts=2
  FIFO Queue : FIFOQueue  Capacity=inf
  Get Attribute : GetAttribute  AttributeName=UoH|Quantity|INFlow  AttributeMissing=Error|Error|Error  AttributeDefaultValue=1|1|1  AttributeTreatAsVector=1|1|1  AttributeSendTiming=After entity departure|After entity departure|After entity departure  EvaluatedDefaultAttributeValue={[];[];[]}
      settings: OutputPortMap=o1,o2,o3
  Set Attribute : SetAttribute  AttributeName=INFlow  AttributeFrom=Signal port  EvaluatedAttributeValue={[]}
  Single Server : SingleServer  ServiceTime=0
  FlowRecord_IN : PMIOPort  Port=1  Side=Right
  FlowRecord_OUT : PMIOPort  Port=2  Side=Right
  INFlow_Signal : PMIOPort  Port=3  Side=Left
  wires:
  Get Attribute/1 -> Calculate_INFlow/1(UoH)
  Calculate_INFlow/1(INFlow_return) -> Set Attribute/1
  Get Attribute/2 -> Calculate_INFlow/2(Quantity)
  Get Attribute/3 -> Calculate_INFlow/3(INFlow)
  connections:
  Entity Combiner/RConn1 -- Get Attribute/LConn1
  Set Attribute/RConn1 -- Entity Splitter/LConn1
  Get Attribute/RConn1 -- Single Server/LConn1
  Single Server/RConn1 -- Set Attribute/LConn1
  FlowRecord_OUT/RConn1 -- Entity Splitter/RConn1
  FlowRecord_IN/RConn1 -- Entity Combiner/LConn1
  Entity Splitter/RConn2 -- Entity Sink/LConn1
  INFlow_Signal/RConn1 -- FIFO Queue/LConn1
  FIFO Queue/RConn1 -- Entity Combiner/LConn2

== system FRNmodel_IMHRC/FastCarton2MPassembly/Calculate_OUTFlow ==
  Calculate_OUTFlow : MATLAB Function  TreatAsAtomicUnit=on
  Entity Combiner : EntityCombiner  NumberInputPorts=2
  Entity Sink : EntitySink
  Entity Splitter : EntitySplitter  NumberOutputPorts=2
  FIFO Queue : FIFOQueue  Capacity=inf
  Get Attribute : GetAttribute  AttributeName=UoH|Quantity|OUTFlow  AttributeMissing=Error|Error|Error  AttributeDefaultValue=1|1|1  AttributeTreatAsVector=1|1|1  AttributeSendTiming=After entity departure|After entity departure|After entity departure  EvaluatedDefaultAttributeValue={[];[];[]}
      settings: OutputPortMap=o1,o2,o3
  Set Attribute : SetAttribute  AttributeName=OUTFlow  AttributeFrom=Signal port  EvaluatedAttributeValue={[]}
  Single Server : SingleServer  ServiceTime=0
  FlowRecord_IN : PMIOPort  Port=1  Side=Left
  FlowRecord_OUT : PMIOPort  Port=2  Side=Left
  OUTFlow_Signal : PMIOPort  Port=3  Side=Right
  wires:
  Get Attribute/1 -> Calculate_OUTFlow/1(UoH)
  Calculate_OUTFlow/1(OUTFlow_return) -> Set Attribute/1
  Get Attribute/2 -> Calculate_OUTFlow/2(Quantity)
  Get Attribute/3 -> Calculate_OUTFlow/3(OUTFlow)
  connections:
  Entity Combiner/RConn1 -- Get Attribute/LConn1
  Set Attribute/RConn1 -- Entity Splitter/LConn1
  Get Attribute/RConn1 -- Single Server/LConn1
  Single Server/RConn1 -- Set Attribute/LConn1
  FlowRecord_OUT/RConn1 -- Entity Splitter/RConn1
  FlowRecord_IN/RConn1 -- Entity Combiner/LConn1
  OUTFlow_Signal/RConn1 -- FIFO Queue/LConn1
  FIFO Queue/RConn1 -- Entity Combiner/LConn2
  Entity Splitter/RConn2 -- Entity Sink/LConn1

== system FRNmodel_IMHRC/FastCarton2MPassembly/FRN_Process ==
  FIFO Queue1 : FIFOQueue
  N-Server : NServer  NumberOfServers=inf  ServiceTime=0
  Flow_IN : PMIOPort  Port=1  Side=Left
  Message_IN : PMIOPort  Port=2  Side=Left
  Flow_OUT : PMIOPort  Port=3  Side=Right
  Message_OUT : PMIOPort  Port=4  Side=Right
  connections:
  FIFO Queue1/RConn1 -- N-Server/LConn1
  Flow_IN/RConn1 -- FIFO Queue1/LConn1
  Flow_OUT/RConn1 -- N-Server/RConn1
  Message_OUT/RConn1 -- Message_IN/RConn1

== system FRNmodel_IMHRC/FastCarton2MPassembly/FlowRecord ==
  Discrete Event Signal to Workspace : simeventslib/SimEvents Sinks/Discrete Event Signal to Workspace  VariableName=INFlow_Metric  SaveFormat=Structure With Time  isMonitorOnly=off  isRecordIC=off
  Discrete Event Signal to Workspace1 : simeventslib/SimEvents Sinks/Discrete Event Signal to Workspace  VariableName=OUTFlow_Metric  SaveFormat=Structure With Time  isMonitorOnly=off  isRecordIC=off
  FIFO Queue : FIFOQueue
  FlowRecord : TimeBasedFunctionCallGenerator  EventGenerationMode=Only at simulation start
  Get Attribute : GetAttribute  AttributeName=OUTFlow|INFlow  AttributeMissing=Error|Error  AttributeDefaultValue=1|1  AttributeTreatAsVector=1|1  AttributeSendTiming=After entity departure|After entity departure  EvaluatedDefaultAttributeValue={[];[]}
      settings: OutputPortMap=o1,o2
  Initialize_FlowRecord : SetAttribute  AttributeName=INFlow|OUTFlow  AttributeFrom=Dialog|Dialog  AttributeValue=[0 0 0 0 0]|[0 0 0 0 0]  AttributeTreatAsVector=1|1  EvaluatedAttributeValue={[0 0 0 0 0];[0 0 0 0 0]}
  New_FlowRecord : EventBasedEntityGenerator  GenerateEntitiesUpon=Function call from port fcn
  Output Switch : OutputSwitch  NumberOutputPorts=2
  Path Combiner1 : PathCombiner
  TO_INFlow : PMIOPort  Port=1  Side=Right
  TO_OUTFlow : PMIOPort  Port=2  Side=Left
  FROM_INFlow : PMIOPort  Port=3  Side=Right
  FROM_OUTFlow : PMIOPort  Port=4  Side=Left
  wires:
  FlowRecord/1 -> New_FlowRecord/1
  Get Attribute/2 -> Discrete Event Signal to Workspace/1
  Get Attribute/1 -> Discrete Event Signal to Workspace1/1
  connections:
  Output Switch/LConn1 -- FIFO Queue/RConn1
  New_FlowRecord/RConn1 -- Initialize_FlowRecord/LConn1
  Initialize_FlowRecord/RConn1 -- Path Combiner1/LConn1
  TO_INFlow/RConn1 -- Output Switch/RConn1
  TO_OUTFlow/RConn1 -- Output Switch/RConn2
  FROM_INFlow/RConn1 -- Path Combiner1/LConn2
  FROM_OUTFlow/RConn1 -- Path Combiner1/LConn3
  Path Combiner1/RConn1 -- Get Attribute/LConn1
  Get Attribute/RConn1 -- FIFO Queue/LConn1
